simulink model "P1FA"  (Simulink 4.00)
settings: Solver=ode45  StartTime=0.0  StopTime=10.0  RelTol=1e-3
libraries: simulink3 x2, dsparch3 x1
settings Model: LastModifiedBy=Administrador  BlockReductionOpt=off

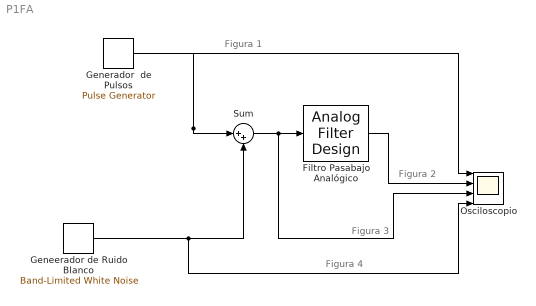
== system P1FA ==
  note: Figura 1
  note: Figura 2
  note: Figura 3
  note: Figura 4
  Filtro Pasabajo Analógico : dsparch3/Analog Filter Design  method=Butterworth  filttype=Lowpass  N=10  Wlo=10  Whi=80  Rp=2  Rs=40
  Geneerador de Ruido Blanco : simulink3/Sources/Band-Limited White Noise  Cov=[0.01]  Ts=0.05  seed=[23341]
  Generador  de Pulsos : simulink3/Sources/Pulse Generator  period=1  duty=50  amplitude=4  start=0
  Osciloscopio : Scope  NumInputPorts=4
      settings: TimeRange=10  YMin=-5~-5~-5~-5  YMax=5~5~5~5  SaveToWorkspace=off  SaveName=ScopeData  LimitDataPoints=on  MaxDataPoints=5000
  Sum : Sum  Inputs=|++  SaturateOnIntegerOverflow=on
  wires:
  Sum/1 -> Osciloscopio/3, Filtro Pasabajo Analógico/1
  Filtro Pasabajo Analógico/1 -> Osciloscopio/2
  Generador  de Pulsos/1 -> Sum/1, Osciloscopio/1
  Geneerador de Ruido Blanco/1 -> Sum/2, Osciloscopio/4
